simulink model "AP_AH"  (R2018a)
settings: Solver=VariableStepAuto  StartTime=0.0  StopTime=S.simtime  RelTol=1e-3
undefined symbols (not defined in the file): kq, S, sigbuilder_block
settings Model: Creator=Can Bekar  LastModifiedBy=Can Bekar
settings DataIOCC: ExternalInput=S.usignal  LoadExternalInput=on  SignalLogging=off  DSMLogging=off

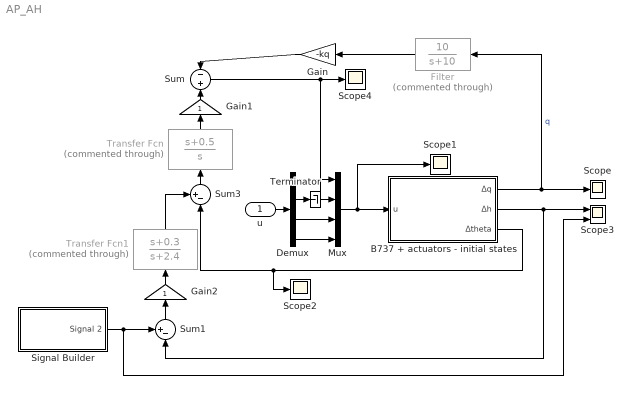
== system AP_AH ==
  u : Inport
  B737 + actuators - initial states : Subsystem
  Demux : Demux
  Filter : TransferFcn  Commented=through  Numerator=[10]  Denominator=[1 10]
  Gain : Gain  Gain=-kq
  Gain1 : Gain
  Gain2 : Gain
  Mux : Mux
  Scope{,1..2,4} (4 alike) : Scope
  Scope3 : Scope  NumInputPorts=2
  Signal Builder : Subsystem  Tag=STV Subsys  LoadFcn=sigbuilder_block('load');  StartFcn=sigbuilder_block('start');  StopFcn=sigbuilder_block('stop');  ClipboardFcn=sigbuilder_block('clipboard');  mask(Sigbuilder block){tuvar=[0:10]}
      mask help: Simulink:masks:SigbuilderBlock_MD
      mask init:
      | if ~strcmp(get_param(bdroot(gcbh),'SimulationStatus'),'stopped') tuvar = sigbuilder_block('maskInit'); end
      settings: CopyFcn=sigbuilder_block('copy');  DeleteFcn=sigbuilder_block('delete');  ModelCloseFcn=sigbuilder_block('modelClose');  PreSaveFcn=sigbuilder_block('preSave');  PauseFcn=sigbuilder_block('pause');  ContinueFcn=sigbuilder_block('continue');  NameChangeFcn=sigbuilder_block('namechange');  OpenFcn=sigbuilder_block('open',[233.25 91.5 964.5 399.75 ]);  CloseFcn=sigbuilder_block('close');
      mask Display: plot(0, 0, 100, 100,[2, 2, 32, 32, 2], [68, 8, 8, 68, 68],[32, 2], [38, 38], [32, 19, 2],[53, 60, 44], [32, 17, 17, 2],[16, 16, 31, 31]);txt = getActiveGroup(gcbh);text(2, 100, txt,'verticalAlignment', 'top');
  Sum : Sum  Inputs=-|+
  Sum1 : Sum  Inputs=+-|
  Sum3 : Sum  Inputs=+-|
  Terminator : Terminator
  Transfer Fcn : TransferFcn  Commented=through  Numerator=[1 0.5]  Denominator=[1 0]
  Transfer Fcn1 : TransferFcn  Commented=through  Numerator=[1 0.3]  Denominator=[1 2.4]
  wires:
  u/1 -> Demux/1
  Mux/1 -> B737 + actuators - initial states/1(u), Scope1/1
  B737 + actuators - initial states/2(Δh) -> Sum1/2, Scope3/1
  Demux/1 -> Mux/1
  Demux/3 -> Mux/3
  Demux/4 -> Mux/4
  B737 + actuators - initial states/1(Δq) -> Filter/1, Scope/1  "q"
  Filter/1 -> Gain/1
  Gain/1 -> Sum/1
  Transfer Fcn/1 -> Gain1/1
  Gain1/1 -> Sum/2
  Sum/1 -> Mux/2, Scope4/1
  Gain2/1 -> Transfer Fcn1/1
  Sum1/1 -> Gain2/1
  Sum3/1 -> Transfer Fcn/1
  Transfer Fcn1/1 -> Sum3/1
  B737 + actuators - initial states/3(Δtheta) -> Scope2/1, Sum3/2
  Signal Builder/1(Signal 2) -> Scope3/2, Sum1/1
  Demux/2 -> Terminator/1

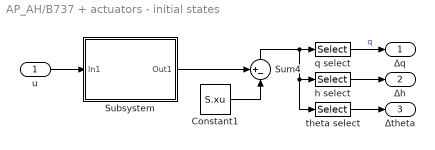
== system AP_AH/B737 + actuators - initial states ==
  u : Inport
  Constant1 : Constant  Value=S.xu
  Subsystem : Subsystem
  Sum4 : Sum  Inputs=+-|
  h select : Selector  InputPortWidth=12  IndexOptions=Index vector (dialog)  Indices=[12]  OutputSizes=1
  q select : Selector  InputPortWidth=12  IndexOptions=Index vector (dialog)  Indices=[8]  OutputSizes=1
  theta select : Selector  InputPortWidth=12  IndexOptions=Index vector (dialog)  Indices=[5]  OutputSizes=1
  Δq : Outport
  Δh : Outport  Port=2
  Δtheta : Outport  Port=3
  wires:
  q select/1 -> Δq/1  "q"
  Sum4/1 -> theta select/1, h select/1, q select/1
  Subsystem/1(Out1) -> Sum4/1
  u/1 -> Subsystem/1(In1)
  Constant1/1 -> Sum4/2
  h select/1 -> Δh/1
  theta select/1 -> Δtheta/1

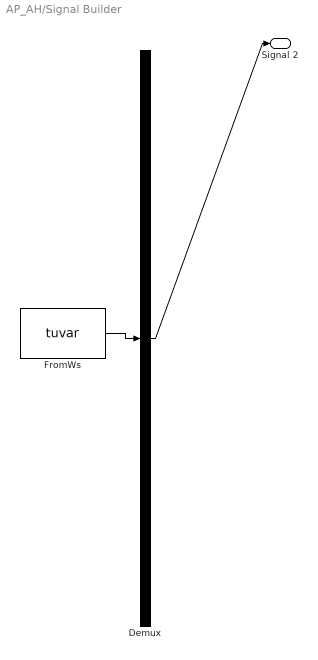
== system AP_AH/Signal Builder ==
  Demux : Demux  Tag=STV Demux  Outputs=1
  FromWs : FromWorkspace  Tag=STV FromWs  VariableName=tuvar  SampleTime=0
      SigBuilderData=|
      | common.afterFinalStr = 'Extrapolate'
      | common.sampleTime = 0
      | dataSet.timeRange = [0 300]
      | dataSet.name = 'Group 1'
      | sbobj.Groups.Name = 'Group 1'
      | sbobj.Groups.Signals.Name = 'Signal 2'
      | sbobj.Groups.Signals.XData = [0 100.5 200 250.5 300]
      | sbobj.Groups.Signals.YData = [0 -3000 -3000 0 0]
      | sbobj.Groups.TimeRange = [0 300]
  Signal 2 : Outport  Tag=STV Outport
  wires:
  FromWs/1 -> Demux/1
  Demux/1 -> Signal 2/1

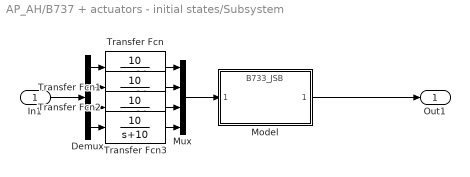
== system AP_AH/B737 + actuators - initial states/Subsystem ==
  In1 : Inport
  Demux : Demux
  Model : ModelReference  ModelNameDialog=B733_JSB  SimulationMode=Normal  ModelReferenceVersion=1.183
  Mux : Mux
  Transfer Fcn{,1..3} (4 alike) : TransferFcn  Numerator=[10]  Denominator=[1 10]
  Out1 : Outport
  wires:
  In1/1 -> Demux/1
  Model/1 -> Out1/1
  Mux/1 -> Model/1
  Transfer Fcn/1 -> Mux/1
  Demux/1 -> Transfer Fcn/1
  Demux/2 -> Transfer Fcn1/1
  Transfer Fcn1/1 -> Mux/2
  Demux/3 -> Transfer Fcn2/1
  Transfer Fcn2/1 -> Mux/3
  Demux/4 -> Transfer Fcn3/1
  Transfer Fcn3/1 -> Mux/4
